simulink model "Ecuacion_diferencial"  (R2023b)
settings: Solver=VariableStepAuto  StartTime=0.0  StopTime=10.0  RelTol=1e-3
InitFcn:
  | R=5.2;
  | L=9.38e-4;
  | J=0.0072;
  | B=3.89e-4;
  | Ra=0.05;
  | km=0.5931;
settings Model: Creator=marqu  LastModifiedBy=marqu

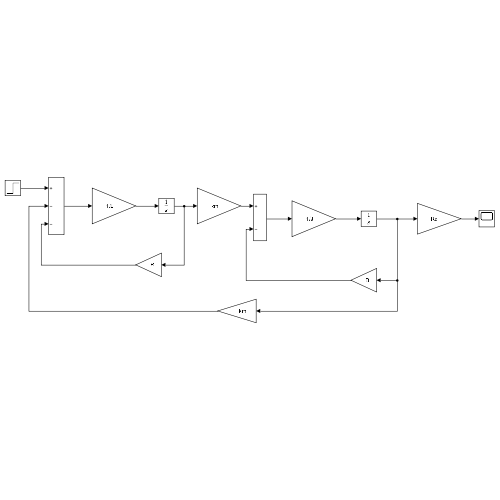
[thumbnail: Simulink's stored preview of the top-level diagram]
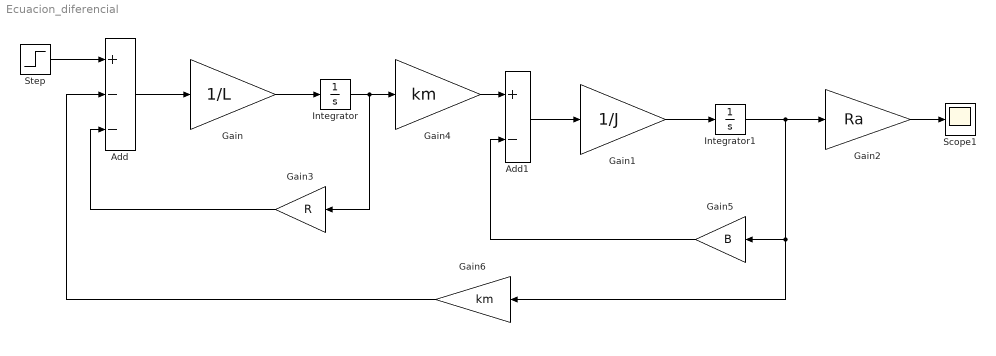
== system Ecuacion_diferencial ==
  Add : Sum  Inputs=+--
  Add1 : Sum  Inputs=+-
  Gain : Gain  Gain=1/L
  Gain1 : Gain  Gain=1/J
  Gain2 : Gain  Gain=Ra
  Gain3 : Gain  Gain=R
  Gain4 : Gain  Gain=km
  Gain5 : Gain  Gain=B
  Gain6 : Gain  Gain=km
  Integrator : Integrator
  Integrator1 : Integrator
  Scope1 : Scope
  Step : Step  After=0.5  SampleTime=0
  wires:
  Step/1 -> Add/1
  Add/1 -> Gain/1
  Gain/1 -> Integrator/1
  Integrator/1 -> Gain3/1, Gain4/1
  Gain4/1 -> Add1/1
  Add1/1 -> Gain1/1
  Gain1/1 -> Integrator1/1
  Integrator1/1 -> Gain6/1, Gain5/1, Gain2/1
  Gain2/1 -> Scope1/1
  Gain3/1 -> Add/3
  Gain6/1 -> Add/2
  Gain5/1 -> Add1/2
